simulink model "processor_ks"  (R2025a)
settings: Solver=VariableStepAuto  StartTime=0.0  StopTime=10.0  RelTol=1e-3
settings Model: Creator=Krutyanjay  LastModifiedBy=Krutyanjay

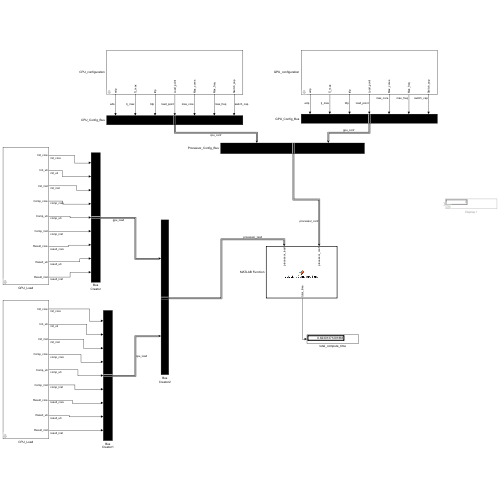
[thumbnail: Simulink's stored preview of the top-level diagram]
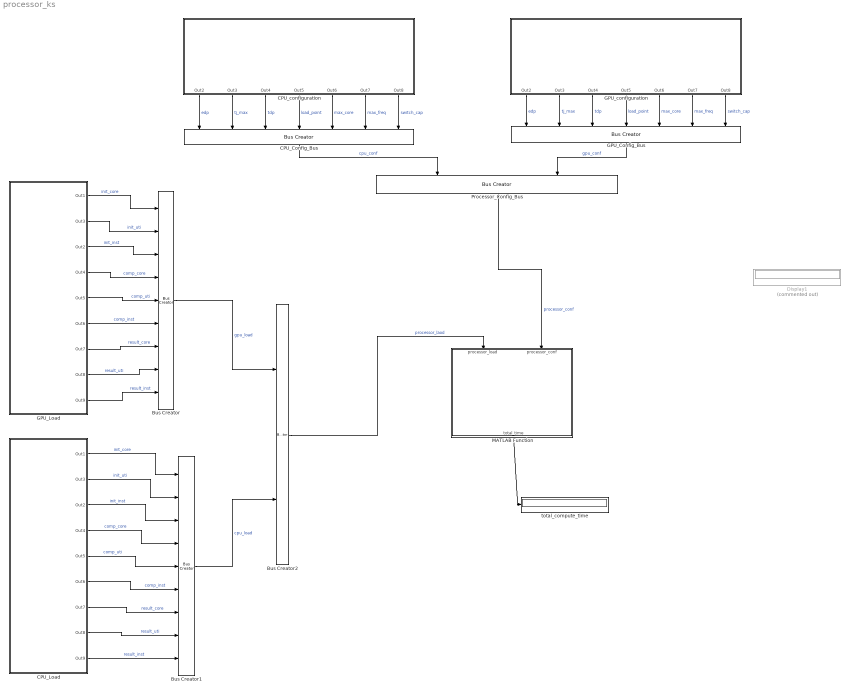
== system processor_ks ==
  Bus Creator : BusCreator  Inputs=9  OutDataTypeStr=Bus: gpu_load
  Bus Creator1 : BusCreator  Inputs=9  OutDataTypeStr=Bus: cpu_load
  Bus Creator2 : BusCreator  Inputs=2  OutDataTypeStr=Bus: processor_load
  CPU_Config_Bus : BusCreator  Inputs=7  OutDataTypeStr=Bus: cpu_conf
  CPU_Load : Subsystem  mask{Init_core=24, Init_uti=0.5, Init_inst=200000, Comp_core=0, Comp_uti=0, Comp_inst=0, Result_core=10, Result_uti=0.5, Result_inst=100000}
      mask prompts: Init_core "Initilization Phase cores"; Init_uti "Total initilization core utilization"; Init_inst "Number of instructions for initilization"; Comp_core "Compute Phase cores"; Comp_uti "Total Compute core utilization"; Comp_inst "Number of isntrutction for compute"; Result_core "Result Phase cores"; Result_uti "Total result core utilization"; Result_inst "Number of instructions for result"
      mask DialogControl saveButton Prompt: Save to CSV
      mask DialogControl loadButton Prompt: Load from CSV
  CPU_configuration : Subsystem  mask{Max_cores=64, Max_freq=2500000000, Switch_cap=31.1, edp=765, tdp=350, Load_point=0.7, Tj_max=100}
      mask prompts: Max_cores "Max Cores"; Max_freq "Max Frequency"; Switch_cap "Active switch capacitance"; Load_point "Load Point"; Tj_max "TjMax"
      mask DialogControl save_button Prompt: Save To CSV
      mask DialogControl load_button Prompt: Load From CSV
  Display1 : Display  Commented=on
  GPU_Config_Bus : BusCreator  Inputs=7  OutDataTypeStr=Bus: gpu_conf
  GPU_Load : Subsystem  mask{Init_core=12, Init_uti=0.1, Init_inst=20000, Comp_core=20000, Comp_uti=0.85, Comp_inst=20000000000000, Result_core=5, Result_uti=0.1, Result_inst=10000}
      mask prompts: Init_core "Initilization Phase cores"; Init_uti "Total initilization core utilization"; Init_inst "Number of instructions for initilization"; Comp_core "Compute Phase cores"; Comp_uti "Total Compute core utilization"; Comp_inst "Number of isntrutction for compute"; Result_core "Result Phase cores"; Result_uti "Total result core utilization"; Result_inst "Number of instructions for result"
      mask DialogControl saveButton Prompt: Save to CSV
      mask DialogControl loadButton Prompt: Load from CSV
  GPU_configuration : Subsystem  mask{Max_cores=16896, Max_freq=1900000000, Switch_cap=184.2, edp=1490, tdp=700, Load_point=0.75, Tj_max=95}
      mask prompts: Max_cores "Max Cores"; Max_freq "Max Frequency"; Switch_cap "Active switch capacitance"; Load_point "Load Point"; Tj_max "TjMax"
      mask DialogControl save_button Prompt: Save To CSV
      mask DialogControl load_button Prompt: Load From CSV
  MATLAB Function : MATLAB Function  TreatAsAtomicUnit=on
  Processor_Config_Bus : BusCreator  Inputs=2  OutDataTypeStr=Bus: processor_conf
  total_compute_time : Display
  wires:
  CPU_configuration/5(Out6) -> CPU_Config_Bus/5  "max_core"
  CPU_configuration/6(Out7) -> CPU_Config_Bus/6  "max_freq"
  CPU_configuration/1(Out2) -> CPU_Config_Bus/1  "edp"
  CPU_configuration/2(Out3) -> CPU_Config_Bus/2  "tj_max"
  CPU_configuration/3(Out4) -> CPU_Config_Bus/3  "tdp"
  CPU_configuration/4(Out5) -> CPU_Config_Bus/4  "load_point"
  CPU_configuration/7(Out8) -> CPU_Config_Bus/7  "switch_cap"
  GPU_configuration/1(Out2) -> GPU_Config_Bus/1  "edp"
  GPU_configuration/2(Out3) -> GPU_Config_Bus/2  "tj_max"
  GPU_configuration/3(Out4) -> GPU_Config_Bus/3  "tdp"
  GPU_configuration/4(Out5) -> GPU_Config_Bus/4  "load_point"
  GPU_configuration/5(Out6) -> GPU_Config_Bus/5  "max_core"
  GPU_configuration/6(Out7) -> GPU_Config_Bus/6  "max_freq"
  GPU_configuration/7(Out8) -> GPU_Config_Bus/7  "switch_cap"
  CPU_Config_Bus/1 -> Processor_Config_Bus/1  "cpu_conf"
  GPU_Config_Bus/1 -> Processor_Config_Bus/2  "gpu_conf"
  GPU_Load/1(Out1) -> Bus Creator/1  "init_core"
  GPU_Load/2(Out3) -> Bus Creator/2  "init_uti"
  CPU_Load/1(Out1) -> Bus Creator1/1  "init_core"
  CPU_Load/2(Out3) -> Bus Creator1/2  "init_uti"
  Bus Creator1/1 -> Bus Creator2/2  "cpu_load"
  Bus Creator/1 -> Bus Creator2/1  "gpu_load"
  Bus Creator2/1 -> MATLAB Function/1(processor_load)  "processor_laod"
  MATLAB Function/1(total_time) -> total_compute_time/1
  GPU_Load/3(Out2) -> Bus Creator/3  "init_inst"
  GPU_Load/4(Out4) -> Bus Creator/4  "comp_core"
  GPU_Load/5(Out5) -> Bus Creator/5  "comp_uti"
  GPU_Load/6(Out6) -> Bus Creator/6  "comp_inst"
  GPU_Load/7(Out7) -> Bus Creator/7  "result_core"
  GPU_Load/8(Out8) -> Bus Creator/8  "result_uti"
  GPU_Load/9(Out9) -> Bus Creator/9  "result_inst"
  CPU_Load/9(Out9) -> Bus Creator1/9  "result_inst"
  CPU_Load/8(Out8) -> Bus Creator1/8  "result_uti"
  CPU_Load/7(Out7) -> Bus Creator1/7  "result_core"
  CPU_Load/6(Out6) -> Bus Creator1/6  "comp_inst"
  CPU_Load/5(Out5) -> Bus Creator1/5  "comp_uti"
  CPU_Load/4(Out4) -> Bus Creator1/4  "comp_core"
  CPU_Load/3(Out2) -> Bus Creator1/3  "init_inst"
  Processor_Config_Bus/1 -> MATLAB Function/2(processor_conf)  "processor_conf"

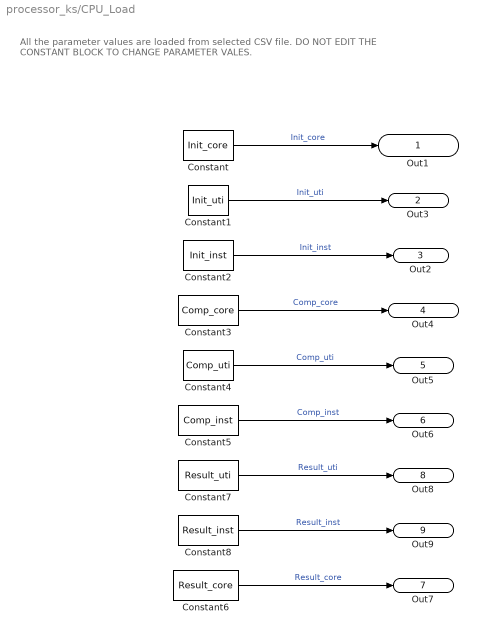
== system processor_ks/CPU_Load ==
  note: All the parameter values are loaded from selected CSV file.
      | DO NOT EDIT THE CONSTANT BLOCK TO CHANGE PARAMETER VALES.
  Constant : Constant  Value=Init_core
  Constant1 : Constant  Value=Init_uti
  Constant2 : Constant  Value=Init_inst
  Constant3 : Constant  Value=Comp_core
  Constant4 : Constant  Value=Comp_uti
  Constant5 : Constant  Value=Comp_inst
  Constant6 : Constant  Value=Result_core
  Constant7 : Constant  Value=Result_uti
  Constant8 : Constant  Value=Result_inst
  Out1 : Outport
  Out3 : Outport  Port=2
  Out2 : Outport  Port=3
  Out4 : Outport  Port=4
  Out5 : Outport  Port=5
  Out6 : Outport  Port=6
  Out7 : Outport  Port=7
  Out8 : Outport  Port=8
  Out9 : Outport  Port=9
  wires:
  Constant7/1 -> Out8/1  "Result_uti"
  Constant5/1 -> Out6/1  "Comp_inst"
  Constant3/1 -> Out4/1  "Comp_core"
  Constant1/1 -> Out3/1  "Init_uti"
  Constant4/1 -> Out5/1  "Comp_uti"
  Constant6/1 -> Out7/1  "Result_core"
  Constant/1 -> Out1/1  "Init_core"
  Constant2/1 -> Out2/1  "Init_inst"
  Constant8/1 -> Out9/1  "Result_inst"

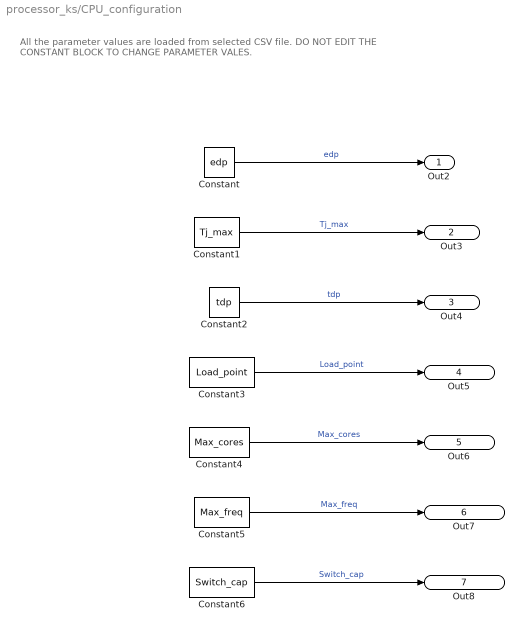
== system processor_ks/CPU_configuration ==
  note: All the parameter values are loaded from selected CSV file.
      | DO NOT EDIT THE CONSTANT BLOCK TO CHANGE PARAMETER VALES.
  Constant : Constant  Value=edp
  Constant1 : Constant  Value=Tj_max
  Constant2 : Constant  Value=tdp
  Constant3 : Constant  Value=Load_point
  Constant4 : Constant  Value=Max_cores
  Constant5 : Constant  Value=Max_freq
  Constant6 : Constant  Value=Switch_cap
  Out2 : Outport
  Out3 : Outport  Port=2
  Out4 : Outport  Port=3
  Out5 : Outport  Port=4
  Out6 : Outport  Port=5
  Out7 : Outport  Port=6
  Out8 : Outport  Port=7
  wires:
  Constant3/1 -> Out5/1  "Load_point"
  Constant5/1 -> Out7/1  "Max_freq"
  Constant4/1 -> Out6/1  "Max_cores"
  Constant/1 -> Out2/1  "edp"
  Constant6/1 -> Out8/1  "Switch_cap"
  Constant1/1 -> Out3/1  "Tj_max"
  Constant2/1 -> Out4/1  "tdp"

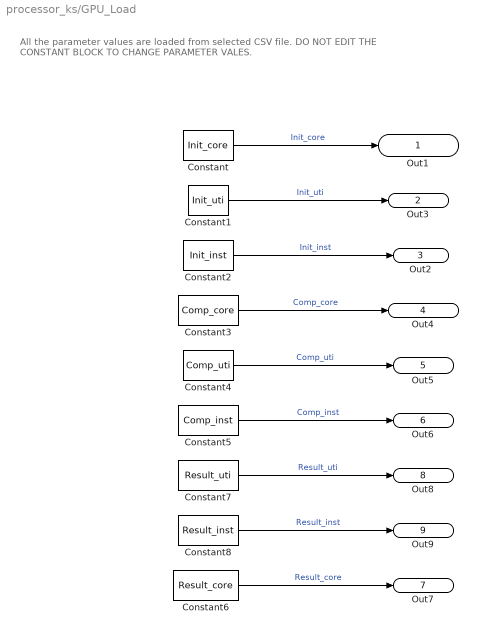
== system processor_ks/GPU_Load ==
  note: All the parameter values are loaded from selected CSV file.
      | DO NOT EDIT THE CONSTANT BLOCK TO CHANGE PARAMETER VALES.
  Constant : Constant  Value=Init_core
  Constant1 : Constant  Value=Init_uti
  Constant2 : Constant  Value=Init_inst
  Constant3 : Constant  Value=Comp_core
  Constant4 : Constant  Value=Comp_uti
  Constant5 : Constant  Value=Comp_inst
  Constant6 : Constant  Value=Result_core
  Constant7 : Constant  Value=Result_uti
  Constant8 : Constant  Value=Result_inst
  Out1 : Outport
  Out3 : Outport  Port=2
  Out2 : Outport  Port=3
  Out4 : Outport  Port=4
  Out5 : Outport  Port=5
  Out6 : Outport  Port=6
  Out7 : Outport  Port=7
  Out8 : Outport  Port=8
  Out9 : Outport  Port=9
  wires:
  Constant7/1 -> Out8/1  "Result_uti"
  Constant5/1 -> Out6/1  "Comp_inst"
  Constant3/1 -> Out4/1  "Comp_core"
  Constant1/1 -> Out3/1  "Init_uti"
  Constant4/1 -> Out5/1  "Comp_uti"
  Constant6/1 -> Out7/1  "Result_core"
  Constant/1 -> Out1/1  "Init_core"
  Constant2/1 -> Out2/1  "Init_inst"
  Constant8/1 -> Out9/1  "Result_inst"

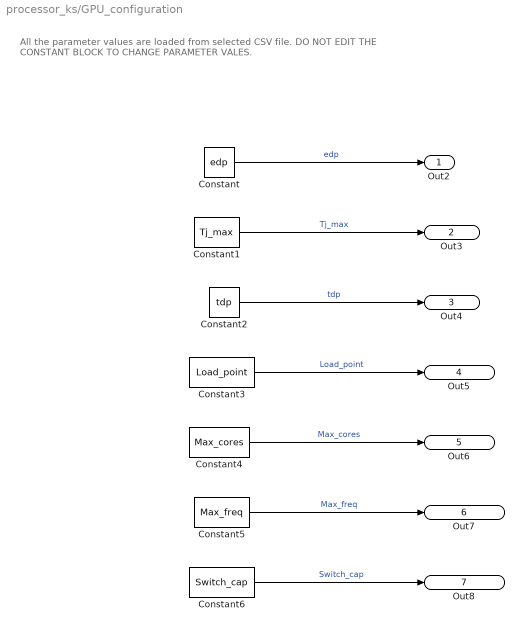
== system processor_ks/GPU_configuration ==
  note: All the parameter values are loaded from selected CSV file.
      | DO NOT EDIT THE CONSTANT BLOCK TO CHANGE PARAMETER VALES.
  Constant : Constant  Value=edp
  Constant1 : Constant  Value=Tj_max
  Constant2 : Constant  Value=tdp
  Constant3 : Constant  Value=Load_point
  Constant4 : Constant  Value=Max_cores
  Constant5 : Constant  Value=Max_freq
  Constant6 : Constant  Value=Switch_cap
  Out2 : Outport
  Out3 : Outport  Port=2
  Out4 : Outport  Port=3
  Out5 : Outport  Port=4
  Out6 : Outport  Port=5
  Out7 : Outport  Port=6
  Out8 : Outport  Port=7
  wires:
  Constant3/1 -> Out5/1  "Load_point"
  Constant5/1 -> Out7/1  "Max_freq"
  Constant4/1 -> Out6/1  "Max_cores"
  Constant/1 -> Out2/1  "edp"
  Constant6/1 -> Out8/1  "Switch_cap"
  Constant1/1 -> Out3/1  "Tj_max"
  Constant2/1 -> Out4/1  "tdp"

== matlab function processor_ks/MATLAB Function ==
  data: processor_load input Bus: processor_load; processor_conf input Bus: processor_conf; total_time output
function total_time = calculateCombinedTime(processor_load, processor_conf)
% This function calculates the combined CPU and GPU compute time.
% It uses the provided logic for individual component time and then
% combines them to account for parallel execution.

% --- A. CPU Performance Calculation ---
% Calculate the time each phase would take on the CPU alone.
% The formula used is from your provided correct logic.
cpu_time_init = processor_load.cpu_load.init_inst / ...
    (min(processor_load.cpu_load.init_core, processor_conf.cpu_conf.max_core) * processor_conf.cpu_conf.max_freq);

% cpu_time_main is now calculated from the input variables.
cpu_time_main = processor_load.cpu_load.comp_inst / ...
    (min(processor_load.cpu_load.comp_core, processor_conf.cpu_conf.max_core) * processor_conf.cpu_conf.max_freq);

cpu_time_result = processor_load.cpu_load.result_inst / ...
    (min(processor_load.cpu_load.result_core, processor_conf.cpu_conf.max_core) * processor_conf.cpu_conf.max_freq);


% --- B. GPU Performance Calculation ---
% Calculate the time each phase would take on the GPU alone.
gpu_time_init = processor_load.gpu_load.init_inst / ...
    (min(processor_load.gpu_load.init_core, processor_conf.gpu_conf.max_core) * processor_conf.gpu_conf.max_freq);

gpu_time_main = processor_load.gpu_load.comp_inst / ...
    (min(processor_load.gpu_load.comp_core, processor_conf.gpu_conf.max_core) * processor_conf.gpu_conf.max_freq);

gpu_time_result = processor_load.gpu_load.result_inst / ...
    (min(processor_load.gpu_load.result_core, processor_conf.gpu_conf.max_core) * processor_conf.gpu_conf.max_freq);


% --- C. Combine Parallel Phase Results ---
% The time for a parallel phase is determined by the SLOWER of the two processors.
time_init   = max(cpu_time_init, gpu_time_init);
time_main   = max(cpu_time_main, gpu_time_main);
time_result = max(cpu_time_result, gpu_time_result);


% --- D. Sum the Phases for the Final Total Time ---
% The total transaction time is the sum of each sequential phase.
total_time = time_init + time_main + time_result;

end
